simulink model "pend_free_sim"  (R2013a)
settings: Solver=ode4  StartTime=0.0  StopTime=tmax-tmin  FixedStep=0.001  RelTol=1e-3
values from neighbouring files (symbols this model uses):
  c2 = 3.2973e-04    (= 0.00032973)    [RotatedPendulumParams.m]    (also in ident_pend.m = p2(2); rotary_ip_lq.m = 1.33e-05)
  g = 9.81    [RotatedPendulumParams.m]    (also in ident_pend.m; rotary_ip_lq.m)
  J2b = p2(1)    [ident_pend.m]    (also in rotary_ip_lq.m = 2.9434e-05)
  l2 = 20e-2    (= 0.2)    [RotatedPendulumParams.m]    (also in ident_pend.m = 0.071; rotary_ip_lq.m = 0.071)
  m2 = 40e-3    (= 0.04)    [RotatedPendulumParams.m]    (also in ident_pend.m = 0.004; rotary_ip_lq.m = 0.004)
  phi20 = A1    [ident_pend.m]
settings Model: Creator=kawata  LastModifiedBy=kawata
settings DataIOCC: SignalLoggingSaveFormat=ModelDataLogs
settings OptimizationCC: ExpressionDepthLimit=2147483647
settings DebuggingCC: FcnCallInpInsideContextMsg=UseLocalSettings
settings GRTTargetCC: CombineOutputUpdateFcns=off  GRTInterface=on

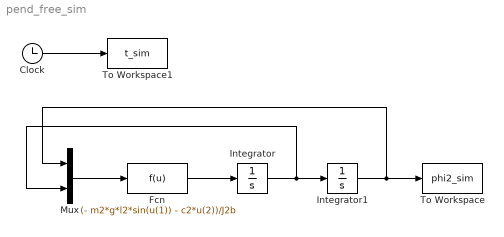
== system pend_free_sim ==
  Clock : Clock
  Fcn : Fcn  Expr=(- m2*g*l2*sin(u(1)) - c2*u(2))/J2b
  Integrator : Integrator
  Integrator1 : Integrator  InitialCondition=phi20
  Mux : Mux  Inputs=2
  To Workspace : ToWorkspace  VariableName=phi2_sim  SampleTime=-1
  To Workspace1 : ToWorkspace  VariableName=t_sim  SampleTime=-1
  wires:
  Clock/1 -> To Workspace1/1
  Integrator1/1 -> To Workspace/1, Mux/1
  Mux/1 -> Fcn/1
  Fcn/1 -> Integrator/1
  Integrator/1 -> Mux/2, Integrator1/1
